simulink model "simulink_FM_MODULATION"  (R2022a)
settings: Solver=VariableStepAuto  StartTime=0.0  StopTime=1  RelTol=1e-3
libraries: commanapbnd3 x2
settings Model: Creator=ASUS  LastModifiedBy=ASUS

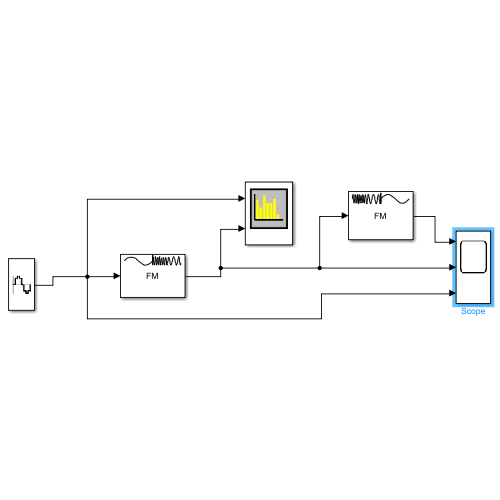
[thumbnail: Simulink's stored preview of the top-level diagram]
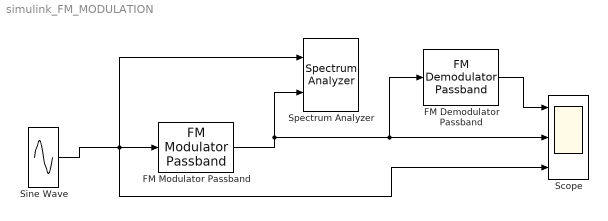
== system simulink_FM_MODULATION ==
  FM Demodulator Passband : commanapbnd3/FM Demodulator Passband  Fc=120  Ph=0  Kc=36  Ho=150
      settings: SourceProductBaseCode=CM
  FM Modulator Passband : commanapbnd3/FM Modulator Passband  Fc=120.000  Ph=0  Kc=36.000
      settings: SourceProductBaseCode=CM
  Scope : Scope  NumInputPorts=3
  Sine Wave : Sin  Amplitude=3  Frequency=12.600  SampleTime=1/10000
  Spectrum Analyzer : SpectrumAnalyzer  NumInputPorts=2
  wires:
  FM Modulator Passband/1 -> Spectrum Analyzer/2, FM Demodulator Passband/1, Scope/2
  Sine Wave/1 -> Scope/3, Spectrum Analyzer/1, FM Modulator Passband/1
  FM Demodulator Passband/1 -> Scope/1
